simulink model "SubsistemaAcondicmientolaser"  (R2023b)
settings: Solver=VariableStepAuto  StartTime=0.0  StopTime=10.0  RelTol=1e-3
settings Model: Creator=manu_  LastModifiedBy=manu_

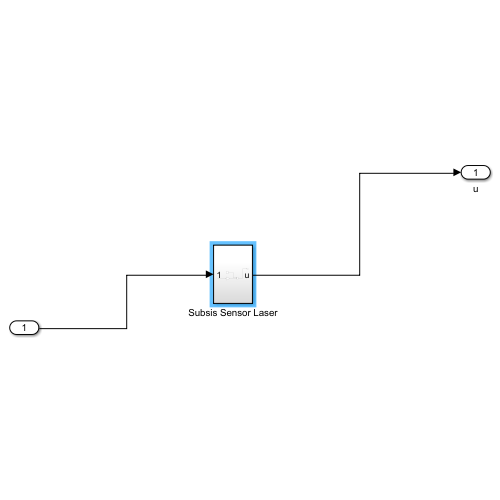
[thumbnail: Simulink's stored preview of the top-level diagram]
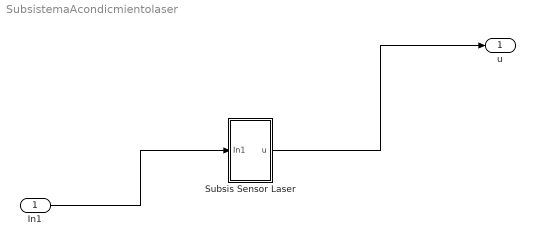
== system SubsistemaAcondicmientolaser ==
  In1 : Inport
  Subsis Sensor Laser : Subsystem
  u : Outport
  wires:
  In1/1 -> Subsis Sensor Laser/1(In1)
  Subsis Sensor Laser/1(u) -> u/1

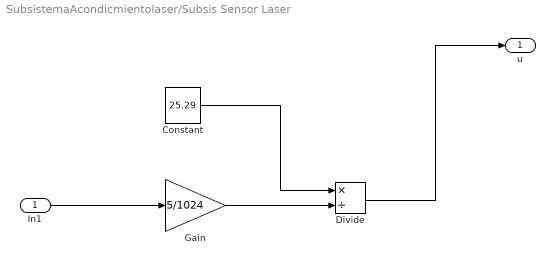
== system SubsistemaAcondicmientolaser/Subsis Sensor Laser ==
  In1 : Inport
  Constant : Constant  Value=25.29
  Divide : Product  Inputs=*/
  Gain : Gain  Gain=5/1024
  u : Outport
  wires:
  In1/1 -> Gain/1
  Divide/1 -> u/1
  Gain/1 -> Divide/2
  Constant/1 -> Divide/1
